simulink model "ACFT"  (R2024a)
settings: Solver=ode1  StartTime=0.0  StopTime=10.0  FixedStep=0.01  RelTol=1e-3  EnableMultiTasking=on
values from neighbouring files (symbols this model uses):
  Inertia = [Ixx 0 -Ixz; 0 Iyy 0; -Ixz 0 Izz]    [initACFT_high.m]
libraries: Aerodynamic x1, Atmospheric x1, EqM x1, Propulsion x1
settings Model: Creator=bruno  LastModifiedBy=hughevr
settings SolverCC: AlgebraicLoopSolver=TrustRegion
settings DataIOCC: ReturnWorkspaceOutputs=off
settings OptimizationCC: LifeSpan=inf
settings DebuggingCC: UnconnectedInputMsg=warning  UnconnectedOutputMsg=warning  UnconnectedLineMsg=warning  SFUnexpectedBacktrackingDiag=warning  SFNoUnconditionalDefaultTransitionDiag=warning  ArithmeticOperatorsInVariantConditions=warning
settings ModelReferenceCC: EnableRefExpFcnMdlSchedulingChecks=on
settings SFSimCC: SimUseLocalCustomCode=off  CustomCodeUndefinedFunction=UseInterfaceOnly
settings RTWCC: RTWUseLocalCustomCode=off  GPUComputeCapability=3.5
settings CodeAppCC: StateflowObjectComments=on
settings GRTTargetCC: TargetLangStandard=C89/C90 (ANSI)
settings ConfigComp: CovMetricSettings=dw  CovSaveCumulativeToWorkspaceVar=on  CovSaveSingleToWorkspaceVar=on  CovExternalEMLEnable=off

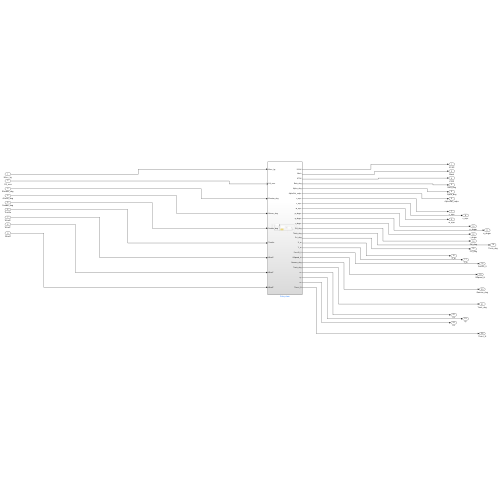
[thumbnail: Simulink's stored preview of the top-level diagram]
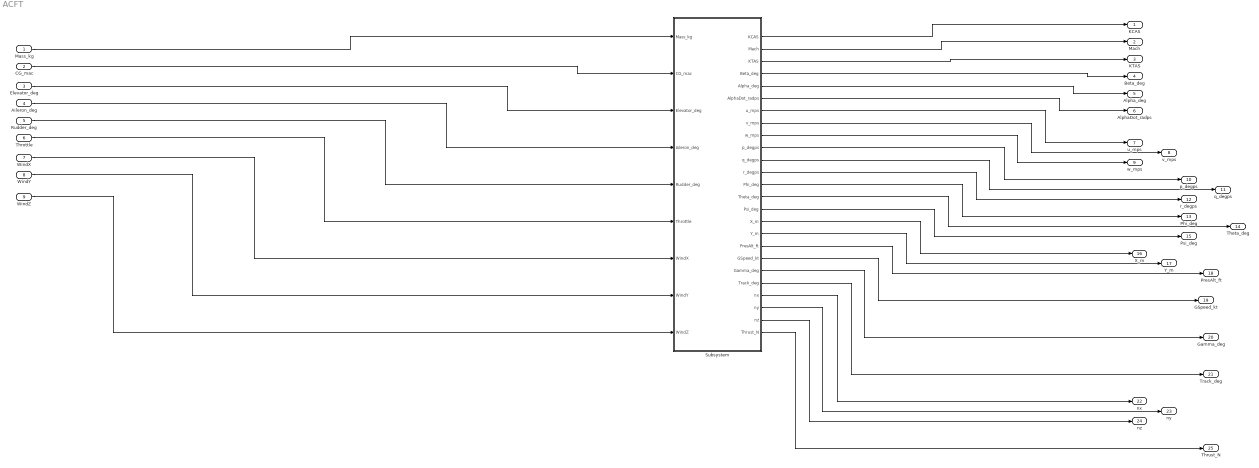
== system ACFT ==
  Mass_kg : Inport  OutDataTypeStr=double
  CG_mac : Inport  Port=2  OutDataTypeStr=double
  Elevator_deg : Inport  Port=3  OutDataTypeStr=double
  Aileron_deg : Inport  Port=4  OutDataTypeStr=double
  Rudder_deg : Inport  Port=5  OutDataTypeStr=double
  Throttle : Inport  Port=6  OutDataTypeStr=double
  WindX : Inport  Port=7  OutDataTypeStr=double
  WindY : Inport  Port=8  OutDataTypeStr=double
  WindZ : Inport  Port=9  OutDataTypeStr=double
  Subsystem : Subsystem
  KCAS : Outport
  Mach : Outport  Port=2
  KTAS : Outport  Port=3
  Beta_deg : Outport  Port=4
  Alpha_deg : Outport  Port=5
  AlphaDot_radps : Outport  Port=6
  u_mps : Outport  Port=7
  v_mps : Outport  Port=8
  w_mps : Outport  Port=9
  p_degps : Outport  Port=10
  q_degps : Outport  Port=11
  r_degps : Outport  Port=12
  Phi_deg : Outport  Port=13
  Theta_deg : Outport  Port=14
  Psi_deg : Outport  Port=15
  X_m : Outport  Port=16
  Y_m : Outport  Port=17
  PresAlt_ft : Outport  Port=18
  GSpeed_kt : Outport  Port=19
  Gamma_deg : Outport  Port=20
  Track_deg : Outport  Port=21
  nx : Outport  Port=22
  ny : Outport  Port=23
  nz : Outport  Port=24
  Thrust_N : Outport  Port=25
  wires:
  Mass_kg/1 -> Subsystem/1(Mass_kg)
  CG_mac/1 -> Subsystem/2(CG_mac)
  Elevator_deg/1 -> Subsystem/3(Elevator_deg)
  Aileron_deg/1 -> Subsystem/4(Aileron_deg)
  Rudder_deg/1 -> Subsystem/5(Rudder_deg)
  Throttle/1 -> Subsystem/6(Throttle)
  WindX/1 -> Subsystem/7(WindX)
  WindY/1 -> Subsystem/8(WindY)
  WindZ/1 -> Subsystem/9(WindZ)
  Subsystem/1(KCAS) -> KCAS/1
  Subsystem/2(Mach) -> Mach/1
  Subsystem/3(KTAS) -> KTAS/1
  Subsystem/4(Beta_deg) -> Beta_deg/1
  Subsystem/5(Alpha_deg) -> Alpha_deg/1
  Subsystem/6(AlphaDot_radps) -> AlphaDot_radps/1
  Subsystem/7(u_mps) -> u_mps/1
  Subsystem/8(v_mps) -> v_mps/1
  Subsystem/9(w_mps) -> w_mps/1
  Subsystem/10(p_degps) -> p_degps/1
  Subsystem/11(q_degps) -> q_degps/1
  Subsystem/12(r_degps) -> r_degps/1
  Subsystem/13(Phi_deg) -> Phi_deg/1
  Subsystem/14(Theta_deg) -> Theta_deg/1
  Subsystem/15(Psi_deg) -> Psi_deg/1
  Subsystem/16(X_m) -> X_m/1
  Subsystem/17(Y_m) -> Y_m/1
  Subsystem/18(PresAlt_ft) -> PresAlt_ft/1
  Subsystem/19(GSpeed_kt) -> GSpeed_kt/1
  Subsystem/20(Gamma_deg) -> Gamma_deg/1
  Subsystem/21(Track_deg) -> Track_deg/1
  Subsystem/22(nx) -> nx/1
  Subsystem/23(ny) -> ny/1
  Subsystem/24(nz) -> nz/1
  Subsystem/25(Thrust_N) -> Thrust_N/1

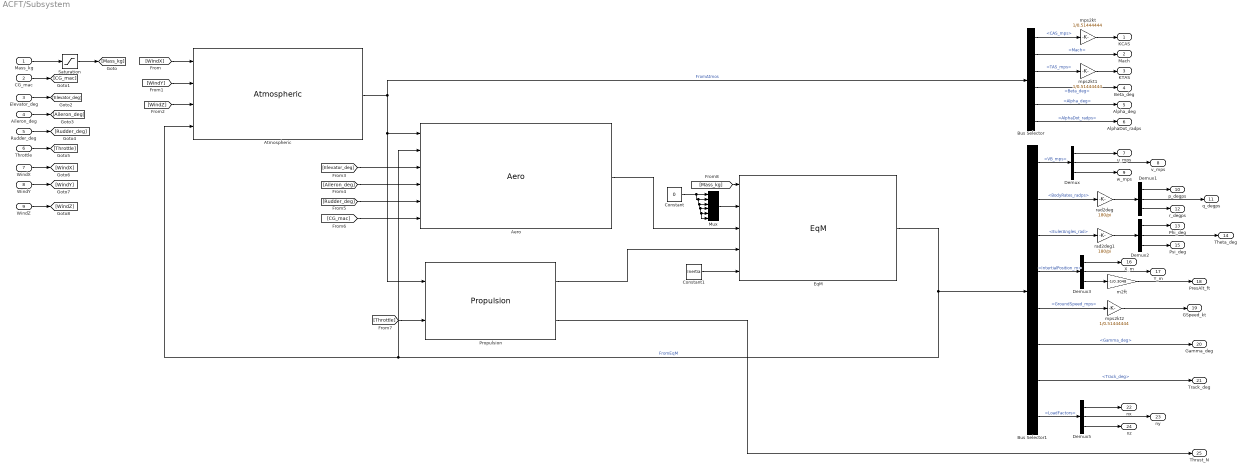
== system ACFT/Subsystem ==
  Mass_kg : Inport  OutDataTypeStr=double
  CG_mac : Inport  Port=2  OutDataTypeStr=double
  Elevator_deg : Inport  Port=3  OutDataTypeStr=double
  Aileron_deg : Inport  Port=4  OutDataTypeStr=double
  Rudder_deg : Inport  Port=5  OutDataTypeStr=double
  Throttle : Inport  Port=6  OutDataTypeStr=double
  WindX : Inport  Port=7  OutDataTypeStr=double
  WindY : Inport  Port=8  OutDataTypeStr=double
  WindZ : Inport  Port=9  OutDataTypeStr=double
  Aero : Aerodynamic/Aero  SystemSampleTime=-1  VariantActivationTime=update diagram  AllowFlexibleInterface=on  Latency=0  AutoFrameSizeCalculation=off
  Atmospheric : Atmospheric/Atmospheric  SystemSampleTime=-1  VariantActivationTime=update diagram  AllowFlexibleInterface=on  Latency=0  AutoFrameSizeCalculation=off
  Bus Selector : BusSelector  OutputSignals=CAS_mps,Mach,TAS_mps,Beta_deg,Alpha_deg,AlphaDot_radps
  Bus Selector1 : BusSelector  OutputSignals=VB_mps,BodyRates_radps,EulerAngles_rad,IntertialPosition_m,GroundSpeed_mps,Gamma_deg,Track_deg,LoadFactors
  Constant : Constant  Value=0  OutDataTypeStr=double
  Constant1 : Constant  Value=Inertia  OutDataTypeStr=double
  Demux{,1..3,5} (5 alike) : Demux  Outputs=3
  EqM : EqM/EqM  SystemSampleTime=-1  VariantActivationTime=update diagram  AllowFlexibleInterface=on  Latency=0  AutoFrameSizeCalculation=off
  Mux : Mux  Inputs=6
  Propulsion : Propulsion/Propulsion  SystemSampleTime=-1  VariantActivationTime=update diagram  AllowFlexibleInterface=on  Latency=0  AutoFrameSizeCalculation=off
  Saturation : Saturate  UpperLimit=inf  LowerLimit=0.1
  m2ft : Gain  Gain=-1/0.3048
  mps2kt : Gain  Gain=1/0.51444444
  mps2kt1 : Gain  Gain=1/0.51444444
  mps2kt2 : Gain  Gain=1/0.51444444
  rad2deg : Gain  Gain=180/pi
  rad2deg1 : Gain  Gain=180/pi
  KCAS : Outport
  Mach : Outport  Port=2
  KTAS : Outport  Port=3
  Beta_deg : Outport  Port=4
  Alpha_deg : Outport  Port=5
  AlphaDot_radps : Outport  Port=6
  u_mps : Outport  Port=7
  v_mps : Outport  Port=8
  w_mps : Outport  Port=9
  p_degps : Outport  Port=10
  q_degps : Outport  Port=11
  r_degps : Outport  Port=12
  Phi_deg : Outport  Port=13
  Theta_deg : Outport  Port=14
  Psi_deg : Outport  Port=15
  X_m : Outport  Port=16
  Y_m : Outport  Port=17
  PresAlt_ft : Outport  Port=18
  GSpeed_kt : Outport  Port=19
  Gamma_deg : Outport  Port=20
  Track_deg : Outport  Port=21
  nx : Outport  Port=22
  ny : Outport  Port=23
  nz : Outport  Port=24
  Thrust_N : Outport  Port=25
  wires:
  Bus Selector/3 -> mps2kt1/1  "<TAS_mps>"
  mps2kt/1 -> KCAS/1
  Bus Selector1/5 -> mps2kt2/1  "<GroundSpeed_mps>"
  Demux2/3 -> Psi_deg/1
  Demux2/1 -> Phi_deg/1
  [CG_mac] -> Aero/6
  Propulsion/1 -> EqM/4
  Atmospheric/1 -> Propulsion/1, Aero/1, Bus Selector/1  "FromAtmos"
  Constant1/1 -> EqM/5
  Bus Selector/2 -> Mach/1  "<Mach>"
  mps2kt1/1 -> KTAS/1
  Demux5/3 -> nz/1
  rad2deg1/1 -> Demux2/1
  [Elevator_deg] -> Aero/3
  [WindZ] -> Atmospheric/3
  [WindX] -> Atmospheric/1
  Rudder_deg/1 -> [Rudder_deg]
  Bus Selector1/2 -> rad2deg/1  "<BodyRates_radps>"
  Mux/1 -> EqM/2
  Bus Selector1/3 -> rad2deg1/1  "<EulerAngles_rad>"
  CG_mac/1 -> [CG_mac]
  WindX/1 -> [WindX]
  Elevator_deg/1 -> [Elevator_deg]
  Demux/3 -> w_mps/1
  Demux/2 -> v_mps/1
  EqM/1 -> Aero/2, Atmospheric/4, Bus Selector1/1  "FromEqM"
  Bus Selector/4 -> Beta_deg/1  "<Beta_deg>"
  [WindY] -> Atmospheric/2
  Bus Selector1/8 -> Demux5/1  "<LoadFactors>"
  WindZ/1 -> [WindZ]
  Aileron_deg/1 -> [Aileron_deg]
  Aero/1 -> EqM/3
  Demux3/2 -> Y_m/1
  Demux3/1 -> X_m/1
  Constant/1 -> Mux/6, Mux/5, Mux/4, Mux/3, Mux/2, Mux/1
  Bus Selector1/6 -> Gamma_deg/1  "<Gamma_deg>"
  Demux3/3 -> m2ft/1
  [Mass_kg] -> EqM/1
  Bus Selector1/1 -> Demux/1  "<VB_mps>"
  Propulsion/2 -> Thrust_N/1
  rad2deg/1 -> Demux1/1
  Demux5/1 -> nx/1
  Demux/1 -> u_mps/1
  Bus Selector/6 -> AlphaDot_radps/1  "<AlphaDot_radps>"
  Demux1/1 -> p_degps/1
  Demux2/2 -> Theta_deg/1
  mps2kt2/1 -> GSpeed_kt/1
  Demux1/3 -> r_degps/1
  Demux5/2 -> ny/1
  Bus Selector/5 -> Alpha_deg/1  "<Alpha_deg>"
  [Throttle] -> Propulsion/2
  WindY/1 -> [WindY]
  [Aileron_deg] -> Aero/4
  Demux1/2 -> q_degps/1
  Bus Selector1/4 -> Demux3/1  "<IntertialPosition_m>"
  [Rudder_deg] -> Aero/5
  m2ft/1 -> PresAlt_ft/1
  Bus Selector1/7 -> Track_deg/1  "<Track_deg>"
  Mass_kg/1 -> Saturation/1
  Throttle/1 -> [Throttle]
  Bus Selector/1 -> mps2kt/1  "<CAS_mps>"
  Saturation/1 -> [Mass_kg]
